simulink model "QUARTERCAR_TPMS"  (R2022a)
settings: Solver=VariableStepAuto  StartTime=0.0  StopTime=10.0  RelTol=1e-3
libraries: simulink x1
settings Model: Creator=sujee  LastModifiedBy=sujee

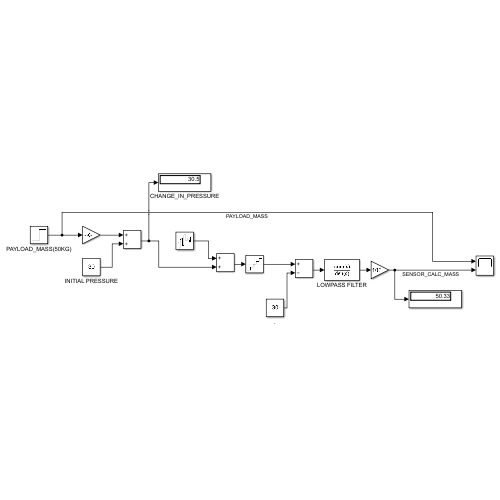
[thumbnail: Simulink's stored preview of the top-level diagram]
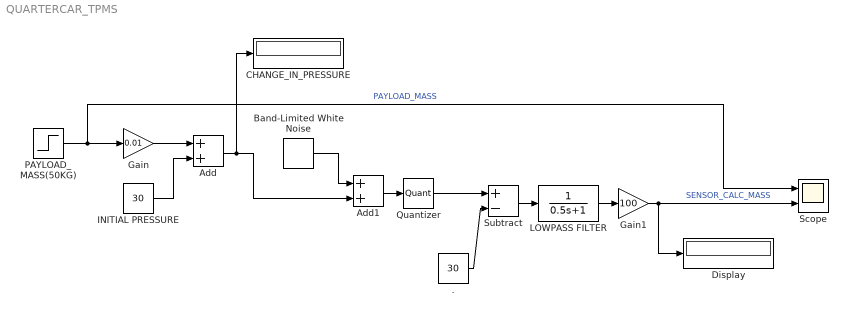
== system QUARTERCAR_TPMS ==
  . : Constant  Value=30
  Add : Sum
  Add1 : Sum
  Band-Limited White Noise : simulink/Sources/Band-Limited White Noise  Cov=[0.0001]  Ts=0.1  seed=[23341]
  CHANGE_IN_PRESSURE : Display
  Display : Display
  Gain : Gain  Gain=0.01
  Gain1 : Gain  Gain=100
  INITIAL PRESSURE : Constant  Value=30
  LOWPASS FILTER : TransferFcn  Denominator=[0.5 1]
  PAYLOAD_MASS(50KG) : Step  Time=2  After=50  SampleTime=0
  Quantizer : Quantizer  QuantizationInterval=0.1  LinearizeAsGain=off
  Scope : Scope  NumInputPorts=2
  Subtract : Sum  Inputs=+-
  wires:
  PAYLOAD_MASS(50KG)/1 -> Scope/1, Gain/1  "PAYLOAD_MASS"
  Gain/1 -> Add/1
  INITIAL PRESSURE/1 -> Add/2
  Band-Limited White Noise/1 -> Add1/1
  Add1/1 -> Quantizer/1
  Add/1 -> CHANGE_IN_PRESSURE/1, Add1/2
  Subtract/1 -> LOWPASS FILTER/1
  Gain1/1 -> Display/1, Scope/2  "SENSOR_CALC_MASS"
  Quantizer/1 -> Subtract/1
  LOWPASS FILTER/1 -> Gain1/1
  ./1 -> Subtract/2
